simulink library "Vehicle_Axle2"  (R2025a)
settings: Solver=VariableStepAuto  StartTime=0.0  StopTime=10.0  RelTol=1e-3
undefined symbols (not defined in the file): Free, Init, RaceFix, RaceSpin, Vehicle
libraries: sm_lib x4, Body_Utilities x1, Brakes_Axle2 x1, Chassis_Axle2 x1, Driveline_Axle2 x1, Power_Systems x1
Description:
  | Component of Simscape Vehicle Templates Library
  | 
  | Copyright 2018-2025 The MathWorks, Inc.
settings Model: Creator=smiller  LastModifiedBy=smiller
settings SolverCC: AlgebraicLoopSolver=TrustRegion
settings DataIOCC: ReturnWorkspaceOutputs=off
settings DebuggingCC: UnconnectedInputMsg=warning  UnconnectedOutputMsg=warning  UnconnectedLineMsg=warning  ArithmeticOperatorsInVariantConditions=warning
settings ModelReferenceCC: EnableRefExpFcnMdlSchedulingChecks=on
settings SFSimCC: CustomCodeUndefinedFunction=UseInterfaceOnly
settings RTWCC: GPUComputeCapability=3.5  DLArmComputeVersion=19.05

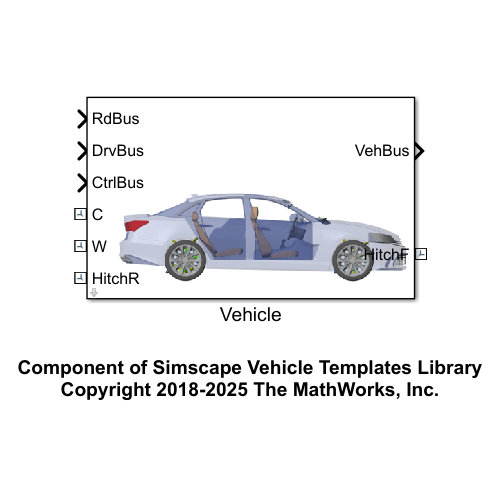
[thumbnail: Simulink's stored preview of the top-level diagram]
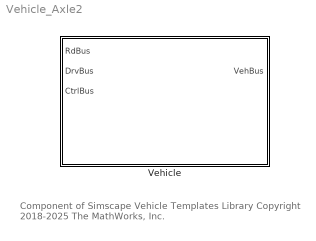
== system Vehicle_Axle2 ==
  note: Component of Simscape Vehicle Templates Library
      | Copyright 2018-2025 The MathWorks, Inc.
  Vehicle : Subsystem  Tag=PublishSubsystem  VariantControl=NS_Con  mask(Vehicle with Two Axles){popup_BodyToWorld=Free, popup_wheel_spin=Free, Vehicle=Vehicle, Init=Init, SpecifyPosTarget=on, veh_index=1, mask_image_name=sm_car_vehicle_hamba_IMAGE.png}
      mask prompts: popup_BodyToWorld "Body To World Connection"; popup_wheel_spin "Wheel Spin"; Vehicle "Vehicle Parameters"; Init "Initial Values"; SpecifyPosTarget "Specify Position Target"; veh_index "Vehicle Index (for tires)"; mask_image_name "Mask Image (string)"
      mask help: Vehicle model with multibody suspension. Initial Values data structure sets initial speed of vehicle and wheels. Set tire index to ensure tire results can be saved independently from other vehicles in the model.
      mask Help: web('sm_car_doc_vehicle.html')
      mask TypeOptions popup_BodyToWorld: Body to World/popup_BodyToWorld
      mask TypeOptions popup_wheel_spin: Wheel Spin/popup_wheel_spin
      mask TypeOptions SpecifyPosTarget: Body to World/SpecifyPosTarget
      mask TypeOptions veh_index: Chassis/veh_index
      mask DialogControl cont_sim Prompt: Config
      mask DialogControl cont_connections Prompt: Lock for KnC Test
      mask Display:
      | % Get image from BodyGeometry.class
      | % (active choice for Body Geometry subsystem)
      | temp_veh_bg_class = lower(get_param([gcb '/Chassis/Body/Body Geometry'],'LabelModeActiveChoice'));
      | 
      | imagestr = (['sm_car_vehicle_' temp_veh_bg_class '.png']);
      | if(~exist(imagestr))
      |     imagestr = ['sm_car_vehicle_axle2_default.png'];
      | end
      | 
      | image(imagestr);

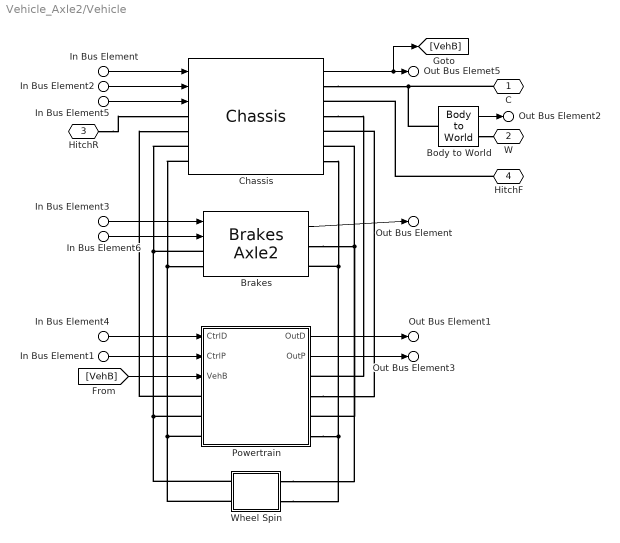
== system Vehicle_Axle2/Vehicle ==
  In Bus Element2 : Inport  PortName=RdBus
  In Bus Element : Inport  Port=2  PortName=DrvBus
  In Bus Element3 : Inport  Port=2  PortName=DrvBus
  In Bus Element6 : Inport  Port=3  PortName=CtrlBus  Element=Brakes
  In Bus Element5 : Inport  Port=3  PortName=CtrlBus  Element=Chassis
  In Bus Element1 : Inport  Port=3  PortName=CtrlBus  Element=Power
  In Bus Element4 : Inport  Port=3  PortName=CtrlBus  Element=Driveline
  Body to World : Body_Utilities/Body to World  VariantControl=Choice  LabelModeActiveChoice=Free  popup_BodyToWorld=Free  SpecifyPosTarget=on
  Brakes : Brakes_Axle2/Brakes Axle2  Tag=PublishSubsystem  VariantControl=Variant1  LabelModeActiveChoice=PedalAbstract_DiscDisc  Brakes=Vehicle.Brakes  VariantLabel=Vehicle.Brakes.class.Value
      settings: AttributesFormatString=%<ActiveVariant>
  Chassis : Chassis_Axle2/Chassis  Tag=PublishSubsystem  VariantControl=Chassis  Chassis=Vehicle.Chassis  Init=Init  mask_image_name=sm_car_vehicle_chassis_hamba_IMAGE.png  veh_index=veh_index
  Powertrain : Subsystem  mask(Powertrain, 2-Axle){Powertrain=Vehicle.Powertrain}
      mask prompts: Powertrain "Powertrain Parameters"
      mask help: Models power source and driveline for two-axle vehicles. The parameters for the selected options are contained in Powertrain data structure.
      mask Display: image('sm_car_vehicle_powertrain_IMAGE.png')
  Wheel Spin : Subsystem  Variant=on  VariantControlMode=label  VariantControl=Choice  LabelModeActiveChoice=Free  mask(Lock / Unlock Wheels){popup_wheel_spin=Free}
      mask prompts: popup_wheel_spin "Wheel Spin"
      mask help: For kinematics and compliance tests, the wheels need to be locked so they cannot spin. Leave unlocked for all other tests.
      mask init:
      | bh = gcb;
      | wspin = get_param(bh,'popup_wheel_spin');
      | set_param(bh,'LabelModeActiveChoice',wspin)
      settings: AttributesFormatString=%<popup_wheel_spin>
      mask TypeOptions popup_wheel_spin: Free | Lock
      mask Display: disp(' ')
  C : PMIOPort  Side=Left
  W : PMIOPort  Port=2  Side=Left
  HitchR : PMIOPort  Port=3  Side=Left
  HitchF : PMIOPort  Port=4  Side=Right
  Out Bus Elemet5 : Outport  VectorParamsAs1DForOutWhenUnconnected=off  PortName=VehBus  Element=Chassis
  Out Bus Element : Outport  VectorParamsAs1DForOutWhenUnconnected=off  PortName=VehBus  Element=Brakes
  Out Bus Element1 : Outport  VectorParamsAs1DForOutWhenUnconnected=off  PortName=VehBus  Element=Driveline
  Out Bus Element2 : Outport  VectorParamsAs1DForOutWhenUnconnected=off  PortName=VehBus  Element=World
  Out Bus Element3 : Outport  VectorParamsAs1DForOutWhenUnconnected=off  PortName=VehBus  Element=Power
  wires:
  [VehB] -> Powertrain/3(VehB)
  Powertrain/2(OutP) -> Out Bus Element3/1
  Powertrain/1(OutD) -> Out Bus Element1/1
  In Bus Element1/1 -> Powertrain/2(CtrlP)
  In Bus Element4/1 -> Powertrain/1(CtrlD)
  In Bus Element3/1 -> Brakes/1
  Body to World/1 -> Out Bus Element2/1
  In Bus Element6/1 -> Brakes/2
  In Bus Element/1 -> Chassis/1
  In Bus Element2/1 -> Chassis/2
  Chassis/1 -> Out Bus Elemet5/1, [VehB]
  Brakes/1 -> Out Bus Element/1
  In Bus Element5/1 -> Chassis/3
  connections:
  Chassis/RConn3 -- Powertrain/RConn1
  Powertrain/RConn2 -- Chassis/RConn4
  Powertrain/LConn1 -- Chassis/LConn2
  HitchF/RConn1 -- Chassis/RConn2
  Powertrain/LConn2 -- Wheel Spin/LConn1 -- Chassis/LConn3 -- Brakes/LConn1
  Powertrain/LConn3 -- Wheel Spin/LConn2 -- Chassis/LConn4 -- Brakes/LConn2
  Body to World/RConn1 -- W/RConn1
  Chassis/RConn1 -- Body to World/LConn1 -- C/RConn1
  HitchR/RConn1 -- Chassis/LConn1
  Brakes/RConn1 -- Wheel Spin/RConn1 -- Powertrain/RConn3 -- Chassis/RConn5
  Powertrain/RConn4 -- Wheel Spin/RConn2 -- Chassis/RConn6 -- Brakes/RConn2

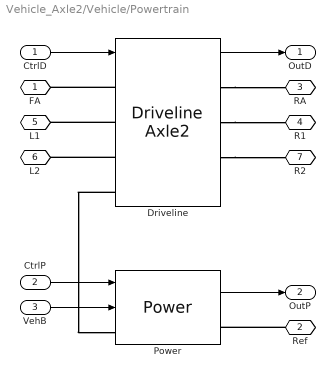
== system Vehicle_Axle2/Vehicle/Powertrain ==
  CtrlD : Inport
  CtrlP : Inport  Port=2
  VehB : Inport  Port=3
  Driveline : Driveline_Axle2/Driveline Axle2  Tag=PublishSubsystem  VariantControl=Shaft  LabelModeActiveChoice=A1_A2_A1Diff_A2Diff  Driveline=Powertrain.Driveline  VariantLabel=Powertrain.Driveline.class.Value
      settings: AttributesFormatString=%<ActiveVariant>
  Power : Power_Systems/Power  VariantControl=Variant1  LabelModeActiveChoice=Ideal_A1_A2  Power=Powertrain.Power  VariantLabel=Powertrain.Power.class.Value
      settings: AttributesFormatString=%<ActiveVariant>
  FA : PMIOPort  Side=Left
  Ref : PMIOPort  Port=2  Side=Right
  RA : PMIOPort  Port=3  Side=Right
  R1 : PMIOPort  Port=4  Side=Right
  L1 : PMIOPort  Port=5  Side=Left
  L2 : PMIOPort  Port=6  Side=Left
  R2 : PMIOPort  Port=7  Side=Right
  OutD : Outport  VectorParamsAs1DForOutWhenUnconnected=off
  OutP : Outport  Port=2  VectorParamsAs1DForOutWhenUnconnected=off
  wires:
  VehB/1 -> Power/2
  CtrlP/1 -> Power/1
  Power/1 -> OutP/1
  CtrlD/1 -> Driveline/1
  Driveline/1 -> OutD/1
  connections:
  Driveline/LConn3 -- L2/RConn1
  Driveline/RConn3 -- R2/RConn1
  Driveline/RConn2 -- R1/RConn1
  Driveline/LConn2 -- L1/RConn1
  Driveline/LConn4 -- Power/LConn1
  Driveline/RConn1 -- RA/RConn1
  Ref/RConn1 -- Power/RConn1
  Driveline/LConn1 -- FA/RConn1

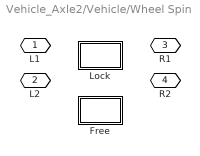
== system Vehicle_Axle2/Vehicle/Wheel Spin ==
  Free : Subsystem  VariantControl=Free
  Lock : Subsystem  VariantControl=Lock
  L1 : PMIOPort  Side=Left
  L2 : PMIOPort  Port=2  Side=Left
  R1 : PMIOPort  Port=3  Side=Right
  R2 : PMIOPort  Port=4  Side=Right

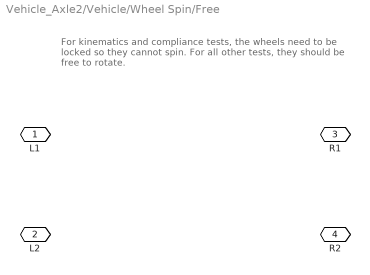
== system Vehicle_Axle2/Vehicle/Wheel Spin/Free ==
  note: For kinematics and compliance tests, the wheels need to be locked so they cannot spin.
      |
      | For all other tests, they should be free to rotate.
  L1 : PMIOPort  Side=Left
  L2 : PMIOPort  Port=2  Side=Left
  R1 : PMIOPort  Port=3  Side=Right
  R2 : PMIOPort  Port=4  Side=Right

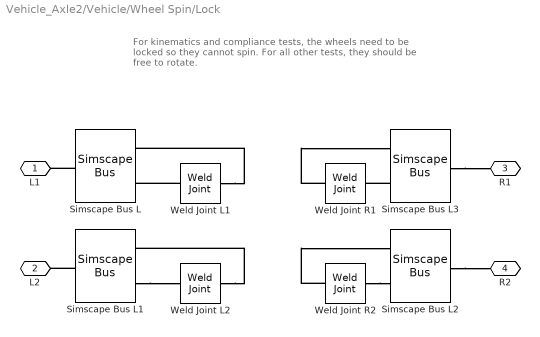
== system Vehicle_Axle2/Vehicle/Wheel Spin/Lock ==
  note: For kinematics and compliance tests, the wheels need to be locked so they cannot spin.
      |
      | For all other tests, they should be free to rotate.
  Simscape Bus L{,1..3} (4 alike) : SimscapeBus  HierarchyStrings=RaceSpin;RaceFix
  Weld Joint L1 : sm_lib/Joints/Weld Joint  JointMode=Normal  CompositeWrenchDir=FollowerOnBase  CompositeWrenchFrame=BaseFrame  SenseConstraintForce=off  SenseConstraintTorque=off  SenseTotalForce=off  SenseTotalTorque=off
  Weld Joint L2 : sm_lib/Joints/Weld Joint  JointMode=Normal  CompositeWrenchDir=FollowerOnBase  CompositeWrenchFrame=BaseFrame  SenseConstraintForce=off  SenseConstraintTorque=off  SenseTotalForce=off  SenseTotalTorque=off
  Weld Joint R1 : sm_lib/Joints/Weld Joint  JointMode=Normal  CompositeWrenchDir=FollowerOnBase  CompositeWrenchFrame=BaseFrame  SenseConstraintForce=off  SenseConstraintTorque=off  SenseTotalForce=off  SenseTotalTorque=off
  Weld Joint R2 : sm_lib/Joints/Weld Joint  JointMode=Normal  CompositeWrenchDir=FollowerOnBase  CompositeWrenchFrame=BaseFrame  SenseConstraintForce=off  SenseConstraintTorque=off  SenseTotalForce=off  SenseTotalTorque=off
  L1 : PMIOPort  Side=Left
  L2 : PMIOPort  Port=2  Side=Left
  R1 : PMIOPort  Port=3  Side=Right
  R2 : PMIOPort  Port=4  Side=Right
  connections:
  Weld Joint L1/LConn1 -- Simscape Bus L/LConn1
  Simscape Bus L/RConn1 -- L1/RConn1
  Weld Joint L1/RConn1 -- Simscape Bus L/LConn2
  Simscape Bus L1/RConn1 -- L2/RConn1
  Simscape Bus L1/LConn2 -- Weld Joint L2/RConn1
  Weld Joint L2/LConn1 -- Simscape Bus L1/LConn1
  Weld Joint R1/LConn1 -- Simscape Bus L3/LConn1
  Weld Joint R2/RConn1 -- Simscape Bus L2/LConn2
  Simscape Bus L3/LConn2 -- Weld Joint R1/RConn1
  Weld Joint R2/LConn1 -- Simscape Bus L2/LConn1
  Simscape Bus L3/RConn1 -- R1/RConn1
  Simscape Bus L2/RConn1 -- R2/RConn1
